simulink model "Sim_Plant_y"  (R2017a)
settings: Solver=ode3  StartTime=0.0  StopTime=10  FixedStep=1/50  RelTol=1e-3  EnableMultiTasking=on
values from neighbouring files (symbols this model uses):
  mQ = 0.5645    [LG_ID_ss_Model.m]
undefined symbols (not defined in the file or in its folder): Kd_y, Kd_z, Kp_y, Kp_z, magnitude
settings Model: Creator=GeoLee  LastModifiedBy=gmh_n
settings DataIOCC: LimitDataPoints=on  SaveFormat=Array
settings OptimizationCC: ExpressionDepthLimit=2147483647  LifeSpan=inf
settings DebuggingCC: UnderspecifiedInitializationDetection=Classic  MergeDetectMultiDrivingBlocksExec=none  SolverPrmCheckMsg=warning  StateNameClashWarn=warning  SFUnexpectedBacktrackingDiag=warning  SFNoUnconditionalDefaultTransitionDiag=warning  SFExecutionAtInitializationDiag=none
settings HardwareCC: ProdBitPerPointer=32  ProdBitPerSizeT=32  ProdBitPerPtrDiffT=32  ProdLargestAtomicFloat=None  ProdIntDivRoundTo=Undefined  ProdEndianess=Unspecified  ProdWordSize=32  ProdHWDeviceType=32-bit Generic
settings ModelReferenceCC: PropagateSignalLabelsOutOfModel=off
settings GRTTargetCC: TargetLangStandard=C89/C90 (ANSI)  GeneratePreprocessorConditionals=Disable all
settings ConfigComp: CovMetricSettings=dw  CovHtmlReporting=on  CovSaveCumulativeToWorkspaceVar=on  CovSaveSingleToWorkspaceVar=on  CovExternalEMLEnable=off

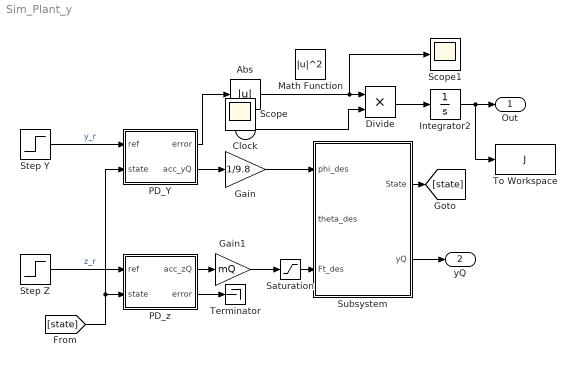
== system Sim_Plant_y ==
  Abs : Abs
  Clock : Clock
  Divide : Product  Inputs=**
  Gain : Gain  Gain=1/9.8
  Gain1 : Gain  Gain=mQ
  Integrator2 : Integrator
  Math Function : Math  Operator=magnitude^2  SaturateOnIntegerOverflow=on
  PD_Y : Subsystem
  PD_z : Subsystem
  Saturation : Saturate  UpperLimit=10  LowerLimit=-0.5645*9.8
  Scope1 : Scope
  Step Y : Step  After=0.2  SampleTime=0
  Step Z : Step  After=0  SampleTime=0
  Subsystem : Subsystem
  Terminator : Terminator
  To Workspace : ToWorkspace  VariableName=J  SampleTime=-1
  Out : Outport
  yQ : Outport  Port=2
  Scope : Scope
  wires:
  Subsystem/1(State) -> [state]
  [state] -> PD_Y/2(state), PD_z/2(state)
  Step Z/1 -> PD_z/1(ref)  "z_r"
  PD_z/1(acc_zQ) -> Gain1/1
  Saturation/1 -> Subsystem/3(Ft_des)
  Integrator2/1 -> To Workspace/1, Out/1
  Divide/1 -> Integrator2/1
  Clock/1 -> Divide/2
  PD_z/2(error) -> Terminator/1
  PD_Y/2(acc_yQ) -> Gain/1
  Step Y/1 -> PD_Y/1(ref)  "y_r"
  PD_Y/1(error) -> Abs/1
  Abs/1 -> Scope1/1, Divide/1
  Gain1/1 -> Saturation/1
  Gain/1 -> Subsystem/1(phi_des)
  Subsystem/2(yQ) -> yQ/1

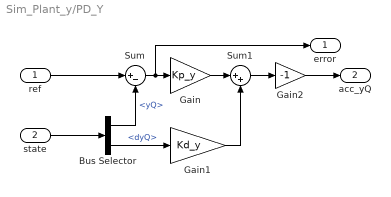
== system Sim_Plant_y/PD_Y ==
  ref : Inport
  state : Inport  Port=2
  Bus Selector : BusSelector  OutputSignals=yQ,dyQ
  Gain : Gain  Gain=Kp_y
  Gain1 : Gain  Gain=Kd_y
  Gain2 : Gain  Gain=-1
  Sum : Sum  Inputs=|+-
  Sum1 : Sum  Inputs=|++
  error : Outport
  acc_yQ : Outport  Port=2
  wires:
  Gain2/1 -> acc_yQ/1
  Gain1/1 -> Sum1/2
  Sum1/1 -> Gain2/1
  Gain/1 -> Sum1/1
  Bus Selector/2 -> Gain1/1  "<dyQ>"
  state/1 -> Bus Selector/1
  ref/1 -> Sum/1
  Bus Selector/1 -> Sum/2  "<yQ>"
  Sum/1 -> error/1, Gain/1

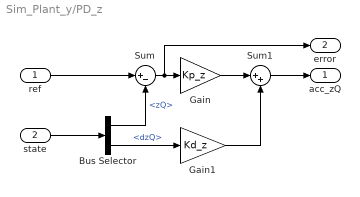
== system Sim_Plant_y/PD_z ==
  ref : Inport
  state : Inport  Port=2
  Bus Selector : BusSelector  OutputSignals=zQ,dzQ
  Gain : Gain  Gain=Kp_z
  Gain1 : Gain  Gain=Kd_z
  Sum : Sum  Inputs=|+-
  Sum1 : Sum  Inputs=|++
  acc_zQ : Outport
  error : Outport  Port=2
  wires:
  Gain1/1 -> Sum1/2
  Sum1/1 -> acc_zQ/1
  Gain/1 -> Sum1/1
  Bus Selector/2 -> Gain1/1  "<dzQ>"
  state/1 -> Bus Selector/1
  Sum/1 -> Gain/1, error/1
  ref/1 -> Sum/1
  Bus Selector/1 -> Sum/2  "<zQ>"

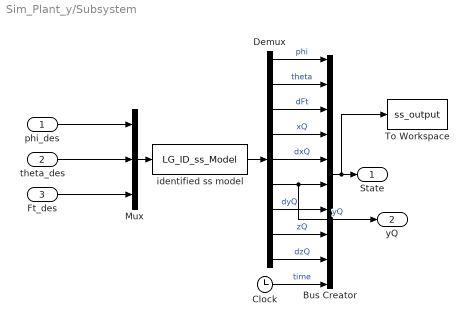
== system Sim_Plant_y/Subsystem ==
  phi_des : Inport
  theta_des : Inport  Port=2
  Ft_des : Inport  Port=3
  Bus Creator : BusCreator  Inputs=10
  Clock : Clock
  Demux : Demux  Outputs=9
  Mux : Mux  Inputs=3
  To Workspace : ToWorkspace  VariableName=ss_output  SampleTime=-1
  identified ss model : S-Function  FunctionName=LG_ID_ss_Model  SFunctionDeploymentMode=off  EnableBusSupport=off
  State : Outport
  yQ : Outport  Port=2
  wires:
  Clock/1 -> Bus Creator/10  "time"
  identified ss model/1 -> Demux/1
  Mux/1 -> identified ss model/1
  Ft_des/1 -> Mux/3
  phi_des/1 -> Mux/1
  theta_des/1 -> Mux/2
  Demux/6 -> yQ/1, Bus Creator/6  "yQ"
  Demux/7 -> Bus Creator/7  "dyQ"
  Demux/4 -> Bus Creator/4  "xQ"
  Demux/9 -> Bus Creator/9  "dzQ"
  Demux/5 -> Bus Creator/5  "dxQ"
  Demux/1 -> Bus Creator/1  "phi"
  Demux/3 -> Bus Creator/3  "dFt"
  Demux/2 -> Bus Creator/2  "theta"
  Demux/8 -> Bus Creator/8  "zQ"
  Bus Creator/1 -> To Workspace/1, State/1
